simulink model "AA_Servoing"  (R2021b)
settings: Solver=ode1  StartTime=0.0  StopTime=inf  FixedStep=0.1  RelTol=1e-3
undefined symbols (not defined in the file): X, Y, Z
libraries: robotlib x7, slpidlib x2, robotmaniplib x2
settings Model: Creator=alessandrini  LastModifiedBy=alessandrini
settings SolverCC: AlgebraicLoopSolver=LineSearch
settings OptimizationCC: EnhancedBackFolding=on  PassReuseOutputArgsThreshold=0  MaxStackSize=64  OptimizeBlockOrder=speed  DifferentSizesBufferReuse=on  OptimizationCustomize=off
settings DebuggingCC: ParameterTunabilityLossMsg=error  SFMachineParentedDataDiag=warning
settings HardwareCC: ProdBitPerPointer=32  ProdBitPerSizeT=32  ProdBitPerPtrDiffT=32  ProdLargestAtomicFloat=None  ProdIntDivRoundTo=Undefined  ProdEndianess=Unspecified  ProdWordSize=32  ProdHWDeviceType=Generic->Unspecified (assume 32-bit Generic)  UseEmbeddedCoderFeatures=off
settings RTWCC: Description=Embedded Coder  SystemTargetFile=ert.tlc  HardwareBoard=Robot Operating System (ROS)  TLCOptions="-aInlineSetEventsForThisBaseRateFcn=TLC_FALSE -aSuppressMultiTaskScheduler=TLC_FALSE  -aRateBasedStepFcn=0"  TemplateMakefile=ert_default_tmf  GenerateReport=on  Toolchain=Catkin  LaunchReport=on  TargetLang=C++
settings CodeAppCC: ForceParamTrailComments=on  OperatorAnnotations=on
settings ERTTargetCC: ERTCustomFileBanners=off  SupportContinuousTime=on  SupportNonInlinedSFcns=on  RemoveResetFunc=off  ModelStepFunctionPrototypeControlCompliant=off

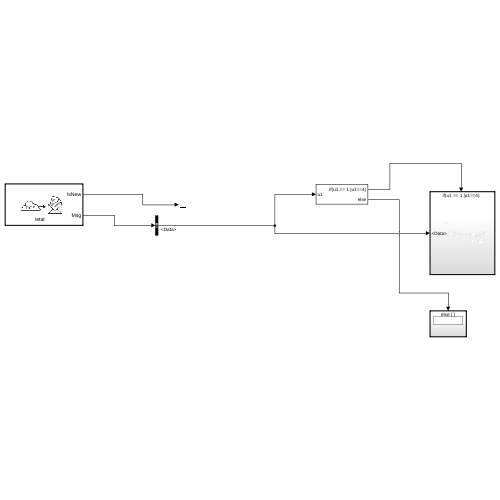
[thumbnail: Simulink's stored preview of the top-level diagram]
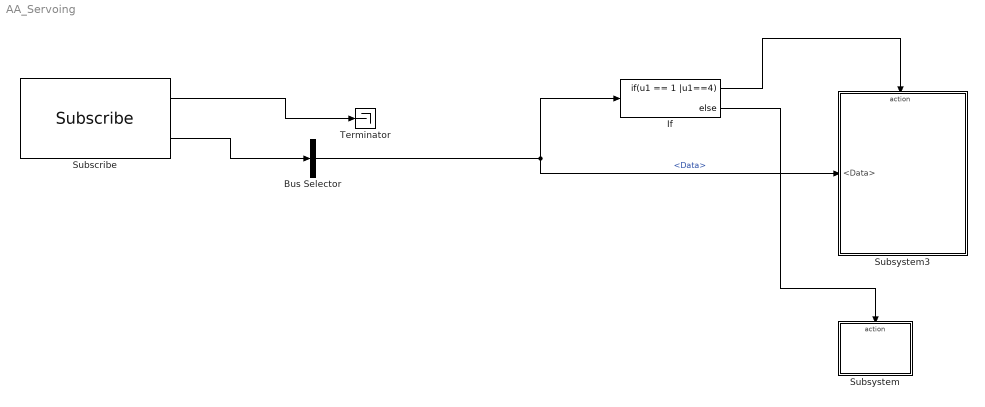
== system AA_Servoing ==
  Bus Selector : BusSelector  OutputSignals=Data
  If : If  IfExpression=u1 == 1 |u1==4
  Subscribe : robotlib/Subscribe  topicSource=Specify your own  topic=/etat  messageType=std_msgs/Int16  SampleTime=-1  legacyBusStruct=off  messageQueueLength=1
  Subsystem : Subsystem
  Subsystem3 : Subsystem
  Terminator : Terminator
  wires:
  Subscribe/2 -> Bus Selector/1
  Subscribe/1 -> Terminator/1
  Bus Selector/1 -> Subsystem3/1(<Data>), If/1  "<Data>"
  If/1 -> Subsystem3/Action
  If/2 -> Subsystem/Action

== system AA_Servoing/Subsystem ==
  Action : ActionPort  InitializeStates=reset  ActionPortLabel=else

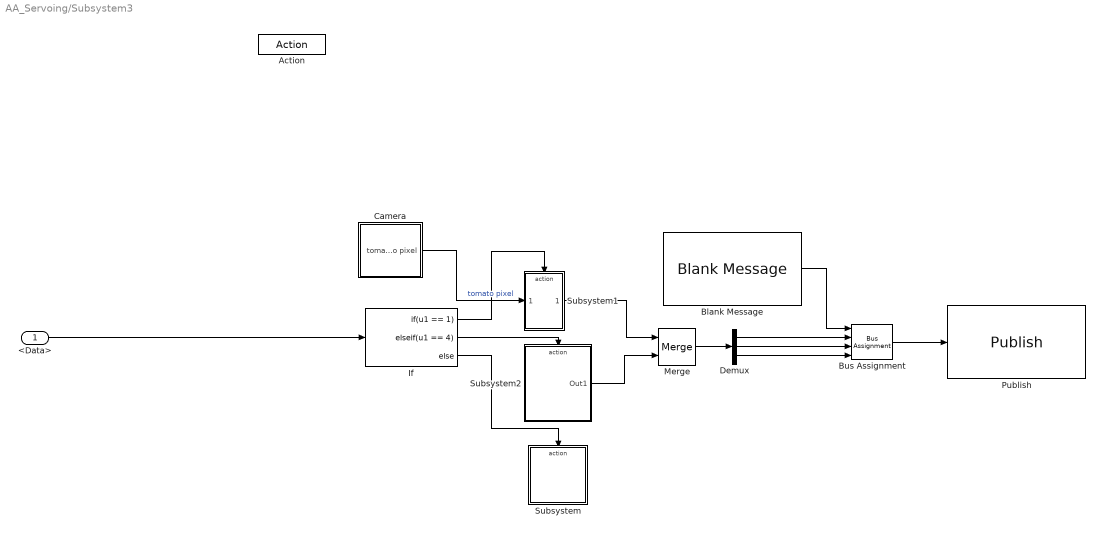
== system AA_Servoing/Subsystem3 ==
  <Data> : Inport
  Action : ActionPort  InitializeStates=reset  ActionPortLabel=if(u1 == 1 |u1==4)
  Blank Message : robotlib/Blank Message  messageClass=Message  entityType=geometry_msgs/Point  messageType=geometry_msgs/Point  SampleTime=inf  legacyBusStruct=off
  Bus Assignment : BusAssignment  AssignedSignals=X,Y,Z
  Camera : Subsystem
  Demux : Demux  Outputs=3
  If : If  IfExpression=u1 == 1  ElseIfExpressions=u1 == 4
  Merge : Merge
  Publish : robotlib/Publish  topicSource=Specify your own  topic=/position_robot  messageType=geometry_msgs/Point  legacyBusStruct=off  messageQueueLength=1
  Subsystem : Subsystem
  Subsystem1 : Subsystem
  Subsystem2 : Subsystem
  wires:
  Subsystem2/1(Out1) -> Merge/2
  If/3 -> Subsystem/Action
  <Data>/1 -> If/1
  Subsystem1/1(Out1) -> Merge/1
  If/1 -> Subsystem1/Action
  Camera/1(tomato pixel) -> Subsystem1/1(tomato pixel)  "tomato pixel"
  If/2 -> Subsystem2/Action
  Bus Assignment/1 -> Publish/1
  Blank Message/1 -> Bus Assignment/1
  Merge/1 -> Demux/1
  Demux/3 -> Bus Assignment/4
  Demux/2 -> Bus Assignment/3
  Demux/1 -> Bus Assignment/2

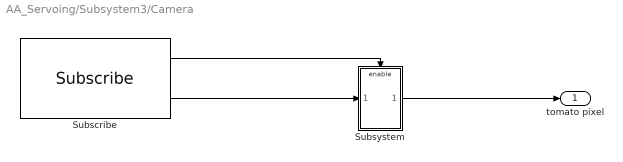
== system AA_Servoing/Subsystem3/Camera ==
  Subscribe : robotlib/Subscribe  topicSource=Specify your own  topic=/tomato_pixels  messageType=geometry_msgs/Point  SampleTime=-1  legacyBusStruct=off  messageQueueLength=1
  Subsystem : Subsystem
  tomato pixel : Outport
  wires:
  Subscribe/2 -> Subsystem/1(In1)
  Subsystem/1(Out1) -> tomato pixel/1
  Subscribe/1 -> Subsystem/Enable

== system AA_Servoing/Subsystem3/Subsystem ==
  Action : ActionPort  InitializeStates=reset  ActionPortLabel=else

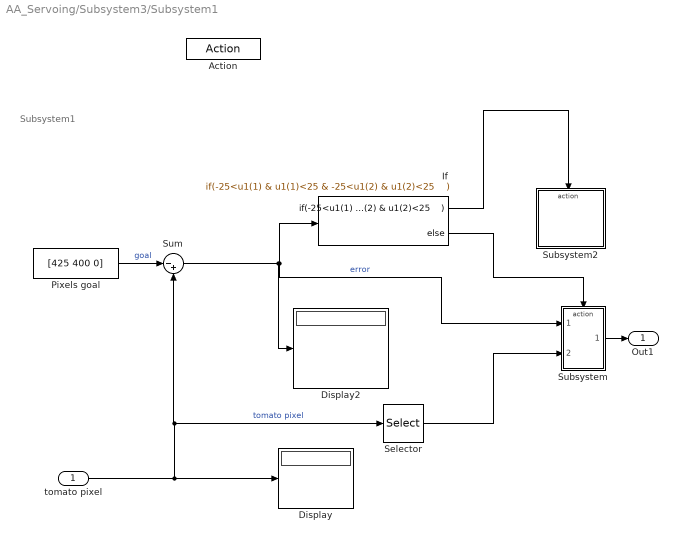
== system AA_Servoing/Subsystem3/Subsystem1 ==
  note: Subsystem1
  tomato pixel : Inport
  Action : ActionPort  InitializeStates=reset  ActionPortLabel=if(u1 == 1)
  Display : Display
  Display2 : Display
  If : If  IfExpression=-25<u1(1) & u1(1)<25 & -25<u1(2) & u1(2)<25
  Pixels goal : Constant  Value=[425 400 0]
  Selector : Selector  InputPortWidth=3  IndexOptions=Index vector (dialog)  Indices=[1]  OutputSizes=1
  Subsystem : Subsystem
  Subsystem2 : Subsystem
  Sum : Sum  Inputs=|-+
  Out1 : Outport
  wires:
  Selector/1 -> Subsystem/2(In2)
  If/1 -> Subsystem2/Action
  If/2 -> Subsystem/Action
  Pixels goal/1 -> Sum/1  "goal"
  tomato pixel/1 -> Sum/2, Selector/1, Display/1  "tomato pixel"
  Sum/1 -> Display2/1, If/1, Subsystem/1(In1)  "error"
  Subsystem/1(Out1) -> Out1/1

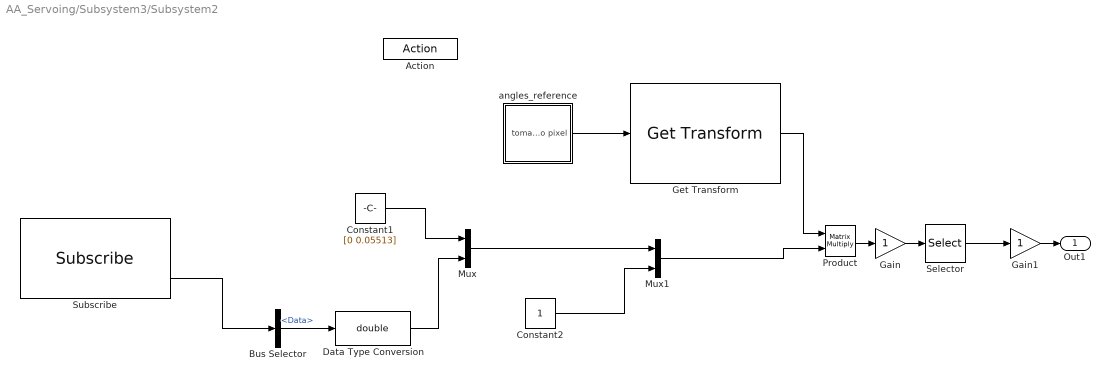
== system AA_Servoing/Subsystem3/Subsystem2 ==
  Action : ActionPort  InitializeStates=reset  ActionPortLabel=elseif(u1 == 4)
  Bus Selector : BusSelector  OutputSignals=Data
  Constant1 : Constant  Value=[0 0.05513]
  Constant2 : Constant
  Data Type Conversion : DataTypeConversion  OutDataTypeStr=double
  Gain : Gain
  Gain1 : Gain
  Get Transform : robotmaniplib/Get Transform  RigidBodyTree=robot  SourceBody=Body6  TargetBody=Base  SimulateUsing=Interpreted execution
  Mux : Mux  Inputs=2
  Mux1 : Mux  Inputs=2
  Product : Product  Multiplication=Matrix(*)
  Selector : Selector  InputPortWidth=4  IndexOptions=Starting index (dialog)  Indices=[1]  OutputSizes=3
  Subscribe : robotlib/Subscribe  topicSource=Specify your own  topic=/depth  messageType=std_msgs/Float32  SampleTime=-1  legacyBusStruct=off  messageQueueLength=1
  angles_reference : Subsystem
  Out1 : Outport
  wires:
  Constant1/1 -> Mux/1
  angles_reference/1(tomato pixel) -> Get Transform/1
  Gain/1 -> Selector/1
  Get Transform/1 -> Product/1
  Selector/1 -> Gain1/1
  Mux/1 -> Mux1/1
  Mux1/1 -> Product/2
  Gain1/1 -> Out1/1
  Product/1 -> Gain/1
  Constant2/1 -> Mux1/2
  Subscribe/2 -> Bus Selector/1
  Bus Selector/1 -> Data Type Conversion/1  "<Data>"
  Data Type Conversion/1 -> Mux/2

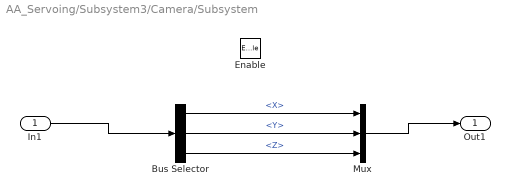
== system AA_Servoing/Subsystem3/Camera/Subsystem ==
  In1 : Inport
  Enable : EnablePort
  Bus Selector : BusSelector  OutputSignals=X,Y,Z
  Mux : Mux  Inputs=3
  Out1 : Outport
  wires:
  In1/1 -> Bus Selector/1
  Bus Selector/2 -> Mux/2  "<Y>"
  Bus Selector/1 -> Mux/1  "<X>"
  Mux/1 -> Out1/1
  Bus Selector/3 -> Mux/3  "<Z>"

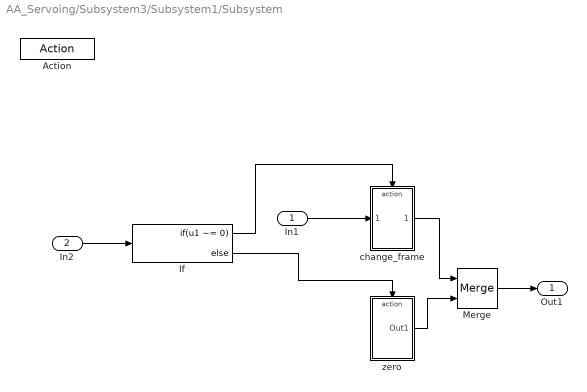
== system AA_Servoing/Subsystem3/Subsystem1/Subsystem ==
  In1 : Inport
  In2 : Inport  Port=2
  Action : ActionPort  InitializeStates=reset  ActionPortLabel=else
  If : If  IfExpression=u1 ~= 0
  Merge : Merge
  change_frame : Subsystem
  zero : Subsystem
  Out1 : Outport
  wires:
  In1/1 -> change_frame/1(In1)
  change_frame/1(Out1) -> Merge/1
  zero/1(Out1) -> Merge/2
  In2/1 -> If/1
  If/1 -> change_frame/Action
  If/2 -> zero/Action
  Merge/1 -> Out1/1

== system AA_Servoing/Subsystem3/Subsystem1/Subsystem2 ==
  Action : ActionPort  InitializeStates=reset  ActionPortLabel="if(-25<u1(1) & u1(1)<25 & -25<u1(2) & u1(2)<25    )"

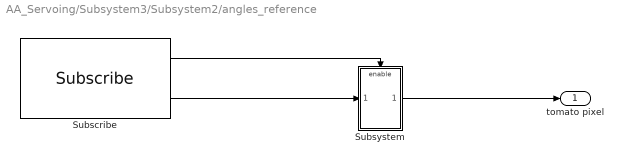
== system AA_Servoing/Subsystem3/Subsystem2/angles_reference ==
  Subscribe : robotlib/Subscribe  topicSource=Specify your own  topic=/angles_joint  messageType=geometry_msgs/Quaternion  SampleTime=-1  legacyBusStruct=off  messageQueueLength=1
  Subsystem : Subsystem
  tomato pixel : Outport
  wires:
  Subscribe/2 -> Subsystem/1(In1)
  Subsystem/1(Out1) -> tomato pixel/1
  Subscribe/1 -> Subsystem/Enable

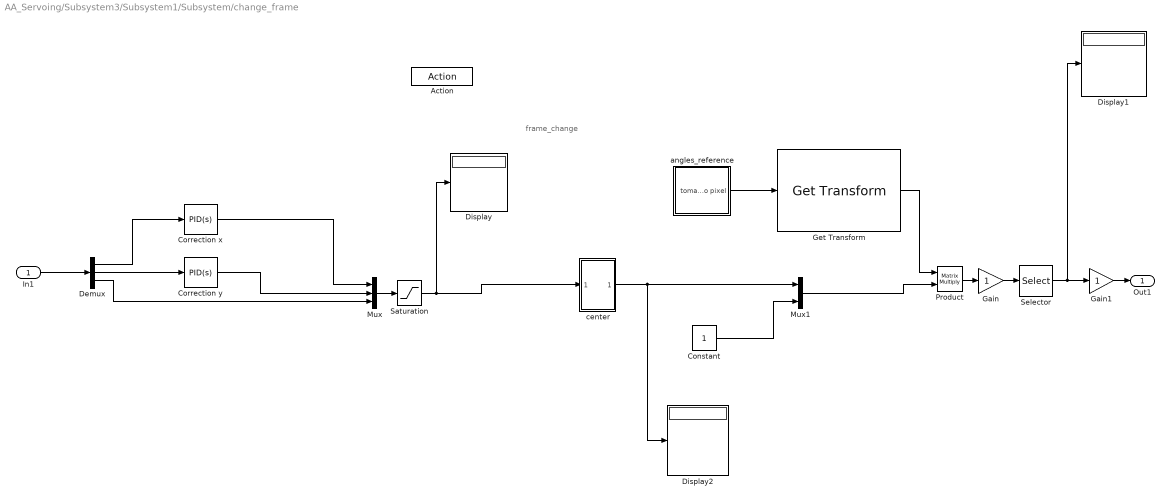
== system AA_Servoing/Subsystem3/Subsystem1/Subsystem/change_frame ==
  note: frame_change
  In1 : Inport
  Action : ActionPort  InitializeStates=reset  ActionPortLabel=if(u1 ~= 0)
  Constant : Constant
  Correction x : slpidlib/PID Controller  Controller=PID  Form=Parallel  TimeDomain=Continuous-time  UseExternalTs=off  SampleTime=-1  IntegratorMethod=Forward Euler  FilterMethod=Forward Euler  ControllerParametersSource=internal  P=0.0001  I=0  D=0  UseFilter=on  N=100  TunerSelectOption=Transfer Function Based (PID Tuner App)  InitialConditionSource=internal  InitialConditionForIntegrator=0  InitialConditionForFilter=0  DifferentiatorICPrevScaledInput=0  ExternalReset=none  TrackingMode=off  Kt=1  LimitOutput=off  SatLimitsSource=internal  UpperSaturationLimit=inf  LowerSaturationLimit=-inf  LinearizeAsGain=on  AntiWindupMode=none  Kb=1  POutMin=[]  POutMax=[]  IOutMin=[]  IOutMax=[]  DOutMin=[]  DOutMax=[]  NOutMin=[]  NOutMax=[]  SumOutMin=[]  SumOutMax=[]  SaturationOutMin=[]  SaturationOutMax=[]  PParamMin=[]  PParamMax=[]  IParamMin=[]  IParamMax=[]  DParamMin=[]  DParamMax=[]  NParamMin=[]  NParamMax=[]  KbParamMin=[]  KbParamMax=[]  KtParamMin=[]  KtParamMax=[]  KbOutMin=[]  KbOutMax=[]  KtOutMin=[]  KtOutMax=[]  IntegratorOutMin=[]  IntegratorOutMax=[]  FilterOutMin=[]  FilterOutMax=[]  SumI1OutMin=[]  SumI1OutMax=[]  SumI2OutMin=[]  SumI2OutMax=[]  SumI3OutMin=[]  SumI3OutMax=[]  SumI4OutMin=[]  SumI4OutMax=[]  SumDOutMin=[]  SumDOutMax=[]  DifferentiatorOutMin=[]  DifferentiatorOutMax=[]  FilterDiffOutCoefMin=[]  FilterDiffOutCoefMax=[]  ReciprocalOutMin=[]  ReciprocalOutMax=[]  SumDenOutMin=[]  SumDenOutMax=[]  SumNumOutMin=[]  SumNumOutMax=[]  DivideOutMin=[]  DivideOutMax=[]  UdiffTsProdOutMin=[]  UdiffTsProdOutMax=[]  NTsProdOutMin=[]  NTsProdOutMax=[]  UintegralTsProdOutMin=[]  UintegralTsProdOutMax=[]  UngainTsProdOutMin=[]  UngainTsProdOutMax=[]  IntegratorContinuousStateAttributes=''  IntegratorStateMustResolveToSignalObject=off  IntegratorRTWStateStorageClass=Auto  FilterContinuousStateAttributes=''  FilterStateMustResolveToSignalObject=off  FilterRTWStateStorageClass=Auto  ParallelPVariant=InternalParameters  IdealPVariant=Disabled  IVariant=InternalParameters  DVariant=InternalParameters  IntegratorVariant=Continuous  SatVariant=Disabled  AWVariant=Passthrough  PCopyVariant=Disabled  TRVariant=Disabled  FdbkBlocksVariant=Forward  IdealPFdbkVariant=Disabled  SatFdbkVariant=Disabled  DerivativeFilterVariant=ContFilter  NVariant=InternalParameters  NCopyVariant=Disabled  FilterICVariant=InternalICsFilter  IntegratorICVariant=InternalICs  ExternalResetVariant=Disabled  TRSumVariant=Passthrough  SumFdbkVariant=Disabled  SumVariant=Sum_PID  TsampFilterVariant=InternalTs  TsampNgainVariant=Passthrough  TsampIntegralVariant=Passthrough  ExternalSaturationOutDataTypeStr=Inherit: Same as second input
  Correction y : slpidlib/PID Controller  Controller=PID  Form=Parallel  TimeDomain=Continuous-time  UseExternalTs=off  SampleTime=-1  IntegratorMethod=Forward Euler  FilterMethod=Forward Euler  ControllerParametersSource=internal  P=0.00416799989827474  I=0  D=0  UseFilter=on  N=100  TunerSelectOption=Transfer Function Based (PID Tuner App)  InitialConditionSource=internal  InitialConditionForIntegrator=0  InitialConditionForFilter=0  DifferentiatorICPrevScaledInput=0  ExternalReset=none  TrackingMode=off  Kt=1  LimitOutput=off  SatLimitsSource=internal  UpperSaturationLimit=inf  LowerSaturationLimit=-inf  LinearizeAsGain=on  AntiWindupMode=none  Kb=1  POutMin=[]  POutMax=[]  IOutMin=[]  IOutMax=[]  DOutMin=[]  DOutMax=[]  NOutMin=[]  NOutMax=[]  SumOutMin=[]  SumOutMax=[]  SaturationOutMin=[]  SaturationOutMax=[]  PParamMin=[]  PParamMax=[]  IParamMin=[]  IParamMax=[]  DParamMin=[]  DParamMax=[]  NParamMin=[]  NParamMax=[]  KbParamMin=[]  KbParamMax=[]  KtParamMin=[]  KtParamMax=[]  KbOutMin=[]  KbOutMax=[]  KtOutMin=[]  KtOutMax=[]  IntegratorOutMin=[]  IntegratorOutMax=[]  FilterOutMin=[]  FilterOutMax=[]  SumI1OutMin=[]  SumI1OutMax=[]  SumI2OutMin=[]  SumI2OutMax=[]  SumI3OutMin=[]  SumI3OutMax=[]  SumI4OutMin=[]  SumI4OutMax=[]  SumDOutMin=[]  SumDOutMax=[]  DifferentiatorOutMin=[]  DifferentiatorOutMax=[]  FilterDiffOutCoefMin=[]  FilterDiffOutCoefMax=[]  ReciprocalOutMin=[]  ReciprocalOutMax=[]  SumDenOutMin=[]  SumDenOutMax=[]  SumNumOutMin=[]  SumNumOutMax=[]  DivideOutMin=[]  DivideOutMax=[]  UdiffTsProdOutMin=[]  UdiffTsProdOutMax=[]  NTsProdOutMin=[]  NTsProdOutMax=[]  UintegralTsProdOutMin=[]  UintegralTsProdOutMax=[]  UngainTsProdOutMin=[]  UngainTsProdOutMax=[]  IntegratorContinuousStateAttributes=''  IntegratorStateMustResolveToSignalObject=off  IntegratorRTWStateStorageClass=Auto  FilterContinuousStateAttributes=''  FilterStateMustResolveToSignalObject=off  FilterRTWStateStorageClass=Auto  ParallelPVariant=InternalParameters  IdealPVariant=Disabled  IVariant=InternalParameters  DVariant=InternalParameters  IntegratorVariant=Continuous  SatVariant=Disabled  AWVariant=Passthrough  PCopyVariant=Disabled  TRVariant=Disabled  FdbkBlocksVariant=Forward  IdealPFdbkVariant=Disabled  SatFdbkVariant=Disabled  DerivativeFilterVariant=ContFilter  NVariant=InternalParameters  NCopyVariant=Disabled  FilterICVariant=InternalICsFilter  IntegratorICVariant=InternalICs  ExternalResetVariant=Disabled  TRSumVariant=Passthrough  SumFdbkVariant=Disabled  SumVariant=Sum_PID  TsampFilterVariant=InternalTs  TsampNgainVariant=Passthrough  TsampIntegralVariant=Passthrough  ExternalSaturationOutDataTypeStr=Inherit: Same as second input
  Demux : Demux  Outputs=3
  Display : Display
  Display1 : Display
  Display2 : Display
  Gain : Gain
  Gain1 : Gain
  Get Transform : robotmaniplib/Get Transform  RigidBodyTree=robot  SourceBody=Body6  TargetBody=Base  SimulateUsing=Interpreted execution
  Mux : Mux  Inputs=3
  Mux1 : Mux  Inputs=2
  Product : Product  Multiplication=Matrix(*)
  Saturation : Saturate  UpperLimit=0.0470740000406901  LowerLimit=-0.08201999918619791
  Selector : Selector  InputPortWidth=4  IndexOptions=Starting index (dialog)  Indices=[1]  OutputSizes=3
  angles_reference : Subsystem
  center : Subsystem
  Out1 : Outport
  wires:
  Correction y/1 -> Mux/2
  angles_reference/1(tomato pixel) -> Get Transform/1
  center/1(Out2) -> Display2/1, Mux1/1
  Get Transform/1 -> Product/1
  Correction x/1 -> Mux/1
  Demux/2 -> Correction y/1
  In1/1 -> Demux/1
  Demux/1 -> Correction x/1
  Gain/1 -> Selector/1
  Demux/3 -> Mux/3
  Mux1/1 -> Product/2
  Mux/1 -> Saturation/1
  Constant/1 -> Mux1/2
  Selector/1 -> Display1/1, Gain1/1
  Product/1 -> Gain/1
  Gain1/1 -> Out1/1
  Saturation/1 -> center/1(In1), Display/1

== system AA_Servoing/Subsystem3/Subsystem1/Subsystem/zero ==
  Action : ActionPort  InitializeStates=reset  ActionPortLabel=else
  Constant : Constant  Value=[-0.173 0.05849 0.4076]
  Out1 : Outport
  wires:
  Constant/1 -> Out1/1

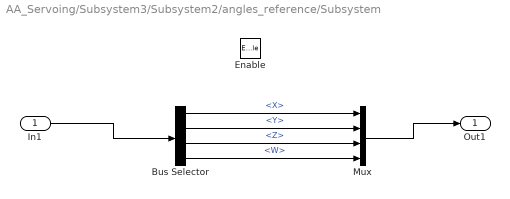
== system AA_Servoing/Subsystem3/Subsystem2/angles_reference/Subsystem ==
  In1 : Inport
  Enable : EnablePort
  Bus Selector : BusSelector  OutputSignals=X,Y,Z,W
  Mux : Mux
  Out1 : Outport
  wires:
  In1/1 -> Bus Selector/1
  Bus Selector/2 -> Mux/2  "<Y>"
  Bus Selector/1 -> Mux/1  "<X>"
  Mux/1 -> Out1/1
  Bus Selector/3 -> Mux/3  "<Z>"
  Bus Selector/4 -> Mux/4  "<W>"

== system AA_Servoing/Subsystem3/Subsystem1/Subsystem/change_frame/angles_reference ==
  Subscribe : robotlib/Subscribe  topicSource=Specify your own  topic=/angles_joint  messageType=geometry_msgs/Quaternion  SampleTime=-1  legacyBusStruct=off  messageQueueLength=1
  Subsystem : Subsystem
  tomato pixel : Outport
  wires:
  Subscribe/2 -> Subsystem/1(In1)
  Subsystem/1(Out1) -> tomato pixel/1
  Subscribe/1 -> Subsystem/Enable

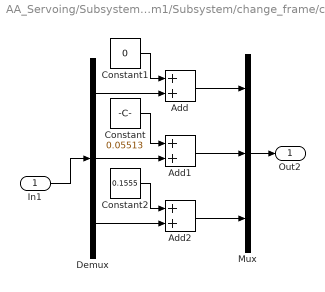
== system AA_Servoing/Subsystem3/Subsystem1/Subsystem/change_frame/center ==
  In1 : Inport
  Add : Sum
  Add1 : Sum
  Add2 : Sum
  Constant : Constant  Value=0.05513
  Constant1 : Constant  Value=0
  Constant2 : Constant  Value=0.1555
  Demux : Demux  Outputs=3
  Mux : Mux  Inputs=3
  Out2 : Outport
  wires:
  In1/1 -> Demux/1
  Demux/2 -> Add1/2
  Demux/1 -> Add/2
  Constant1/1 -> Add/1
  Constant/1 -> Add1/1
  Add1/1 -> Mux/2
  Add/1 -> Mux/1
  Mux/1 -> Out2/1
  Demux/3 -> Add2/2
  Add2/1 -> Mux/3
  Constant2/1 -> Add2/1

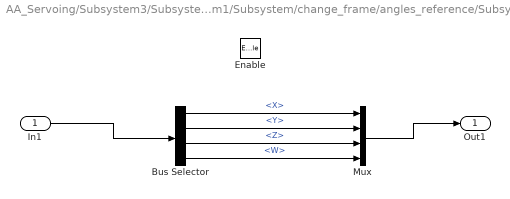
== system AA_Servoing/Subsystem3/Subsystem1/Subsystem/change_frame/angles_reference/Subsystem ==
  In1 : Inport
  Enable : EnablePort
  Bus Selector : BusSelector  OutputSignals=X,Y,Z,W
  Mux : Mux
  Out1 : Outport
  wires:
  In1/1 -> Bus Selector/1
  Bus Selector/2 -> Mux/2  "<Y>"
  Bus Selector/1 -> Mux/1  "<X>"
  Mux/1 -> Out1/1
  Bus Selector/3 -> Mux/3  "<Z>"
  Bus Selector/4 -> Mux/4  "<W>"
